simulink model "deteccion_flancos"  (R2023a)
settings: Solver=FixedStepDiscrete  StartTime=0.0  StopTime=0.4  FixedStep=.0005  RelTol=1e-3
libraries: simulink x7
settings Model: Creator=giohp  LastModifiedBy=Nacho Andrade

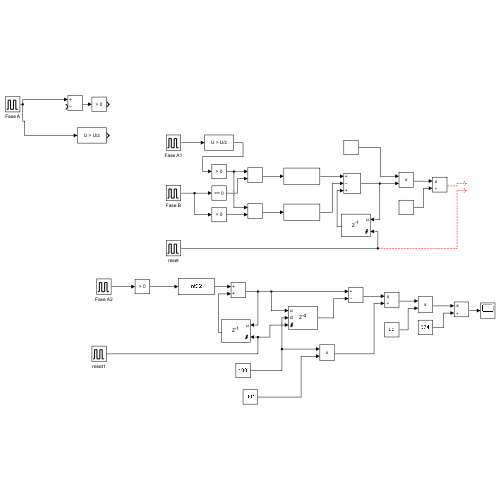
[thumbnail: Simulink's stored preview of the top-level diagram]
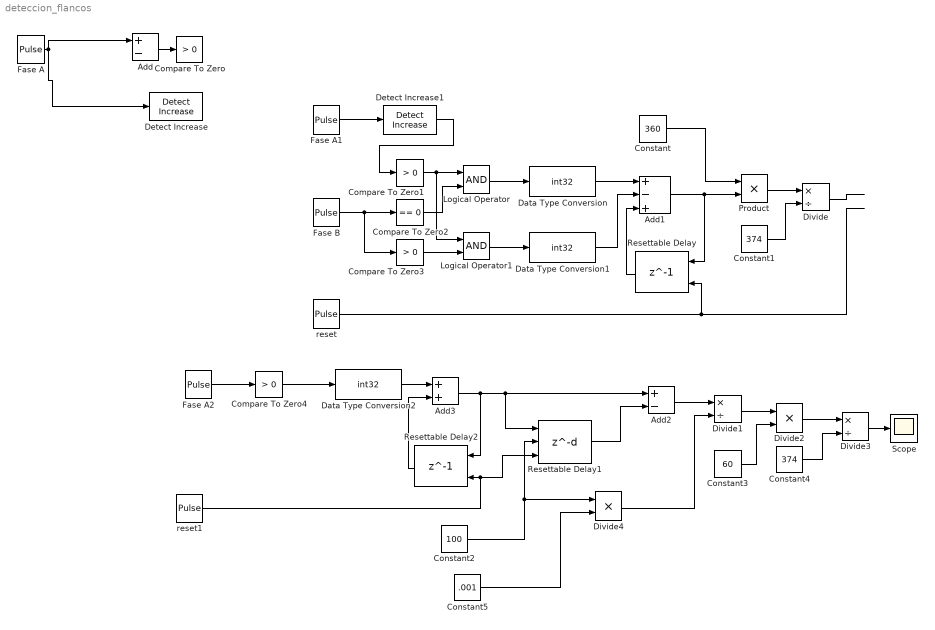
== system deteccion_flancos ==
  Add : Sum  Inputs=+-
  Add1 : Sum  Inputs=+-+
  Add2 : Sum  Inputs=+-
  Add3 : Sum
  Compare To Zero{,1,3..4} (4 alike) : simulink/Logic and Bit Operations/Compare To Zero  relop=>  OutDataTypeStr=boolean
  Compare To Zero2 : simulink/Logic and Bit Operations/Compare To Zero  relop===  OutDataTypeStr=boolean
  Constant : Constant  Value=360
  Constant1 : Constant  Value=374
  Constant2 : Constant  Value=100
  Constant3 : Constant  Value=60
  Constant4 : Constant  Value=374
  Constant5 : Constant  Value=.001
  Data Type Conversion : DataTypeConversion  OutDataTypeStr=int32  SaturateOnIntegerOverflow=off  RndMeth=Floor
  Data Type Conversion1 : DataTypeConversion  OutDataTypeStr=int32  SaturateOnIntegerOverflow=off  RndMeth=Floor
  Data Type Conversion2 : DataTypeConversion  OutDataTypeStr=int32  SaturateOnIntegerOverflow=off  RndMeth=Floor
  Detect Increase : simulink/Logic and Bit Operations/Detect Increase  vinit=0.0  OutDataTypeStr=boolean
  Detect Increase1 : simulink/Logic and Bit Operations/Detect Increase  vinit=0.0  OutDataTypeStr=boolean
  Divide : Product  Inputs=*/
  Divide1 : Product  Inputs=*/
  Divide2 : Product  Inputs=**
  Divide3 : Product  Inputs=*/
  Divide4 : Product  Inputs=**
  Fase A : DiscretePulseGenerator  PulseType=Time based  Amplitude=5  Period=.002  PulseWidth=50
  Fase A1 : DiscretePulseGenerator  PulseType=Time based  Amplitude=5  Period=.002  PulseWidth=50
  Fase A2 : DiscretePulseGenerator  PulseType=Time based  Amplitude=5  Period=.001  PulseWidth=50
  Fase B : DiscretePulseGenerator  PulseType=Time based  Amplitude=5  Period=.002  PulseWidth=50  PhaseDelay=.0005
  Logical Operator : Logic  AllPortsSameDT=off  OutDataTypeStr=boolean
  Logical Operator1 : Logic  AllPortsSameDT=off  OutDataTypeStr=boolean
  Product : Product
  Resettable Delay : Delay  DelayLength=1  ExternalReset=Rising
      settings: InputPortMap=u0,r5
  Resettable Delay1 : Delay  DelayLengthSource=Input port  DelayLength=100  DelayLengthUpperLimit=1000  ExternalReset=Rising
      settings: InputPortMap=u0,p1,r5
  Resettable Delay2 : Delay  DelayLength=1  ExternalReset=Rising
      settings: InputPortMap=u0,r5
  Scope : Scope
  reset : DiscretePulseGenerator  PulseType=Time based  Amplitude=5  Period=.01  PulseWidth=5
  reset1 : DiscretePulseGenerator  PulseType=Time based  Amplitude=5  Period=.01  PulseWidth=5
  wires:
  Fase A/1 -> Add/1, Detect Increase/1
  Add/1 -> Compare To Zero/1
  Compare To Zero1/1 -> Logical Operator1/1, Logical Operator/1
  Fase B/1 -> Compare To Zero3/1, Compare To Zero2/1
  Compare To Zero2/1 -> Logical Operator/2
  Compare To Zero3/1 -> Logical Operator1/2
  Fase A1/1 -> Detect Increase1/1
  Detect Increase1/1 -> Compare To Zero1/1
  Add1/1 -> Resettable Delay/1, Product/2
  Resettable Delay/1 -> Add1/3
  Data Type Conversion/1 -> Add1/1
  Logical Operator/1 -> Data Type Conversion/1
  Logical Operator1/1 -> Data Type Conversion1/1
  Data Type Conversion1/1 -> Add1/2
  Constant/1 -> Product/1
  Product/1 -> Divide/1
  Constant1/1 -> Divide/2
  Divide/1 -> ?
  reset/1 -> Resettable Delay/2
  Divide1/1 -> Divide2/1
  Divide2/1 -> Divide3/1
  Fase A2/1 -> Compare To Zero4/1
  Compare To Zero4/1 -> Data Type Conversion2/1
  Constant3/1 -> Divide2/2
  Constant4/1 -> Divide3/2
  Data Type Conversion2/1 -> Add3/1
  Add3/1 -> Resettable Delay2/1, Resettable Delay1/1, Add2/1
  Resettable Delay2/1 -> Add3/2
  Resettable Delay1/1 -> Add2/2
  Constant2/1 -> Resettable Delay1/2, Divide4/1
  Constant5/1 -> Divide4/2
  Add2/1 -> Divide1/1
  Divide4/1 -> Divide1/2
  Divide3/1 -> Scope/1
  reset1/1 -> Resettable Delay1/3, Resettable Delay2/2
